simulink model "spiBitbang_MainClockDistr_v2_back"  (R2013b)
settings: Solver=FixedStepDiscrete  StartTime=0.0  StopTime=5e-4  FixedStep=Ts  RelTol=1e-3
model workspace (MAT data in the model file):
  Ts = 1e-06
undefined symbols (not defined in the file or in its folder): High, periSam, sampleTime, sigbuilder_block
libraries: simulink_extras x46, simulink x11, dspswit3 x8, dspsnks4 x1
settings Model: Creator=mainster  LastModifiedBy=mainster
settings ConfigurationSet: Description=SimMechanics 2G

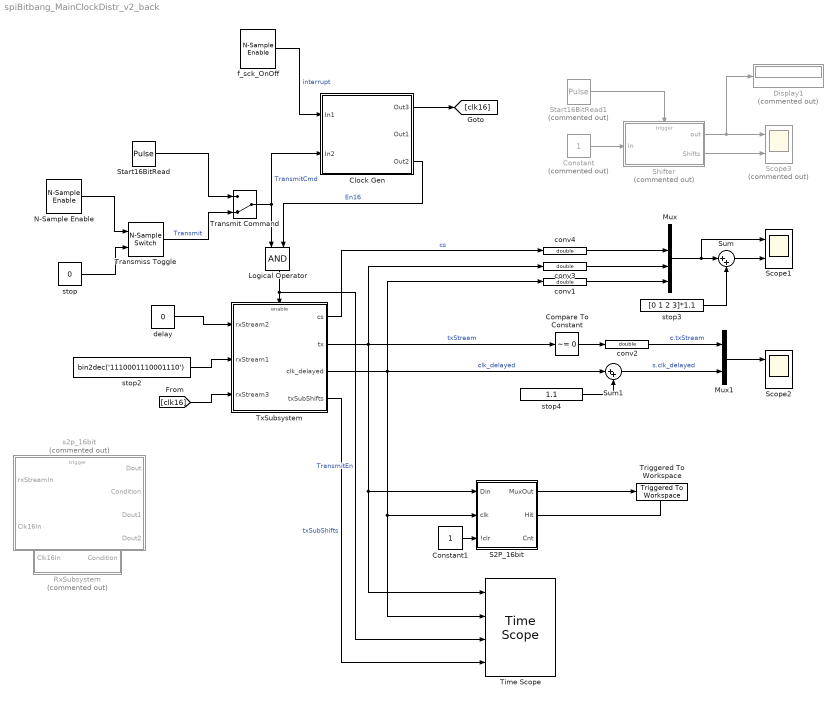
== system spiBitbang_MainClockDistr_v2_back ==
  Clock Gen : Subsystem
  Compare To Constant : simulink/Logic and Bit Operations/Compare To Constant  relop=~=  const=0  OutDataTypeStr=boolean
  Constant : Constant  Commented=on
  Constant1 : Constant  SampleTime=sampleTime
  Display1 : Display  Commented=on
  Logical Operator : Logic  AllPortsSameDT=off  OutDataTypeStr=boolean
  Mux : Mux
  Mux1 : Mux  Inputs=2
  N-Sample Enable : dspswit3/N-Sample Enable  N=20  ActiveLevel=High (1)  reset=off  TriggerType=Rising edge  Ts=-1  DataType=Logical
  RxSubsystem : Subsystem  Commented=on  TreatAsAtomicUnit=on
  S2P_16bit : Subsystem
  Scope1 : Scope  NumInputPorts=2
      settings: ShowLegends=on  TimeRange=0.0015  YMin=-0.2~-0.2  YMax=5~15
  Scope2 : Scope  NumInputPorts=2
      settings: ShowLegends=on  YMin=-0.2~-0.2  YMax=5~15  SaveName=ScopeData4
  Scope3 : Scope  Commented=on  NumInputPorts=2
      settings: ShowLegends=on  TimeRange=0.0015  YMin=-0.2~-0.2  YMax=5~15  SaveName=ScopeData3
  Shifter : Subsystem  Commented=on  TreatAsAtomicUnit=on
  Start16BitRead : DiscretePulseGenerator  Period=400  PulseWidth=35  PhaseDelay=20  SampleTime=Ts
  Start16BitRead1 : DiscretePulseGenerator  Commented=on  Period=100  PulseWidth=50  SampleTime=Ts
  Sum : Sum  Inputs=|++  LockScale=on
  Sum1 : Sum  Inputs=|++  LockScale=on
  Time Scope : TimeScope  NumInputPorts=4  DefaultConfigurationName=spbscopes.TimeScopeBlockCfg
      settings: CopyFcn=scopeextensions.ScopeBlock.onCoreBlockCopy(gcbh);  DeleteFcn=scopeextensions.ScopeBlock.callback(gcbh, 'onBlockDelete');  PreSaveFcn=scopeextensions.ScopeBlock.callback(gcbh, 'onModelSave');  NameChangeFcn=scopeextensions.ScopeBlock.callback(gcbh, 'onBlockRename');  DestroyFcn=scopeextensions.ScopeBlock.onBlockDestroy(gcbh)  CloseFcn=scopeextensions.ScopeBlock.callback(gcbh, 'onBlockClose');  PreDeleteFcn=scopeextensions.ScopeBlock.callback(gcbh, 'onBlockPreDelete');
  Transmiss Toggle : dspswit3/N-Sample Switch  N=250  reset=off  TriggerType=Rising edge  Ts=-1
  Transmit Command : ManualSwitch  CurrentSetting=0
  Triggered To Workspace : dspsnks4/Triggered To Workspace  TriggerType=Rising edge  VariableName=outDffShift  Buffer=1000  Save2DMode=2-D array (concatenate along first dimension)
      settings: FixptAsFi=off
  TxSubsystem : Subsystem
  conv{1..4} (4 alike) : DataTypeConversion  OutDataTypeStr=double  LockScale=on
  delay : Constant  Value=0  SampleTime=-1
  f_sck_OnOff : dspswit3/N-Sample Enable  N=1  ActiveLevel=High (1)  reset=off  TriggerType=Falling edge  Ts=-1  DataType=Boolean
  s2p_16bit : Subsystem  Commented=on
  stop : Constant  Value=0  OutDataTypeStr=Inherit: Inherit via back propagation  SampleTime=-1
  stop2 : Constant  Value=bin2dec('1110001110001110')  OutDataTypeStr=uint16  SampleTime=-1
  stop3 : Constant  Value=[0 1 2 3]*1.1  SampleTime=-1
  stop4 : Constant  Value=1.1  SampleTime=-1
  wires:
  f_sck_OnOff/1 -> Clock Gen/1(In1)  "interrupt"
  Sum/1 -> Scope1/2
  Mux/1 -> Scope1/1, Sum/1
  N-Sample Enable/1 -> Transmiss Toggle/1
  stop/1 -> Transmiss Toggle/2
  Transmit Command/1 -> Logical Operator/1, Clock Gen/2(In2)  "TransmitCmd"
  Transmiss Toggle/1 -> Transmit Command/2  "Transmit"
  Start16BitRead/1 -> Transmit Command/1
  Clock Gen/1(Out3) -> [clk16]
  delay/1 -> TxSubsystem/1(rxStream2)
  [clk16] -> TxSubsystem/3(rxStream3)
  stop2/1 -> TxSubsystem/2(rxStream1)
  stop3/1 -> Sum/2
  TxSubsystem/1(cs) -> conv4/1  "cs"
  conv1/1 -> Mux/4
  Start16BitRead1/1 -> Shifter/Trigger
  Constant/1 -> Shifter/1(In)
  Shifter/1(out) -> Display1/1, Scope3/1
  Shifter/2(Shifts) -> Scope3/2
  TxSubsystem/2(tx) -> Time Scope/1, S2P_16bit/1(Din), conv3/1, Compare To Constant/1  "txStream"
  TxSubsystem/3(clk_delayed) -> conv1/1, Time Scope/2, S2P_16bit/2(clk), Sum1/1  "clk_delayed"
  stop4/1 -> Sum1/2
  Sum1/1 -> Mux1/2  "s.clk_delayed"
  conv3/1 -> Mux/3
  conv4/1 -> Mux/2
  Compare To Constant/1 -> conv2/1
  Mux1/1 -> Scope2/1
  conv2/1 -> Mux1/1  "c.txStream"
  S2P_16bit/1(MuxOut) -> Triggered To Workspace/1
  Constant1/1 -> S2P_16bit/3(!clr)
  S2P_16bit/2(Hit) -> Triggered To Workspace/Trigger
  TxSubsystem/4(txSubShifts) -> Time Scope/4  "txSubShifts"
  Clock Gen/3(Out2) -> Logical Operator/2  "En16"
  Logical Operator/1 -> Time Scope/3, TxSubsystem/Enable  "TransmitEn"

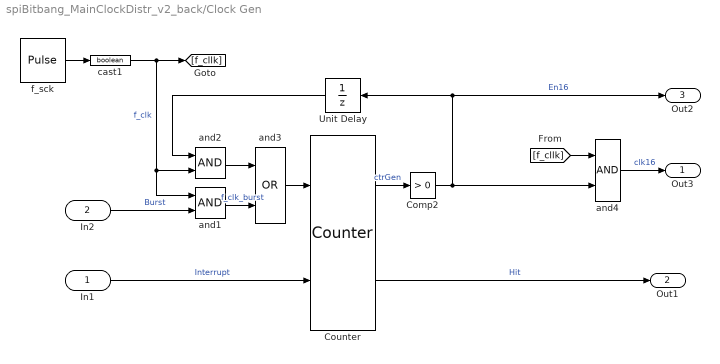
== system spiBitbang_MainClockDistr_v2_back/Clock Gen ==
  In1 : Inport
  In2 : Inport  Port=2
  Comp2 : simulink/Logic and Bit Operations/Compare To Constant  relop=>  const=0  OutDataTypeStr=boolean
  Counter : dspswit3/Counter  Direction=Up  CountEvent=Rising edge  CounterSize=User defined  MaxCount=16  InitialCount=0  Output=Count and Hit  HitValue=periSam/4  ResetInput=on  SamplesPerFrame=1  Ts=1  CntDtype=double  HitDtype=Logical
  Unit Delay : UnitDelay  SampleTime=-1
  and1 : Logic  AllPortsSameDT=off  OutDataTypeStr=boolean
      settings: AttributesFormatString=%<Tag>
  and2 : Logic  AllPortsSameDT=off  OutDataTypeStr=boolean
      settings: AttributesFormatString=%<Tag>
  and3 : Logic  Operator=OR  AllPortsSameDT=off  OutDataTypeStr=boolean
      settings: AttributesFormatString=%<Tag>
  and4 : Logic  AllPortsSameDT=off  OutDataTypeStr=boolean
      settings: AttributesFormatString=%<Tag>
  "cast1 " : DataTypeConversion  OutDataTypeStr=boolean
  f_sck : DiscretePulseGenerator  Period=periSam  PulseWidth=periSam/2  SampleTime=Ts
      settings: AttributesFormatString=|
      | Period =%<Period>
      | sTime=%<SampleTime>
      | Delay=%<PhaseDelay>
  Out3 : Outport
  Out1 : Outport  Port=2
  Out2 : Outport  Port=3
  wires:
  "cast1 "/1 -> and1/1, and2/2, [f_cllk]  "f_clk"
  f_sck/1 -> "cast1 "/1
  Comp2/1 -> Out2/1, Unit Delay/1, and4/2  "En16"
  Counter/1 -> Comp2/1  "ctrGen"
  In1/1 -> Counter/2  "Interrupt"
  In2/1 -> and1/2  "Burst"
  and3/1 -> Counter/1
  and4/1 -> Out3/1  "clk16"
  and1/1 -> and3/2  "f_clk_burst"
  and2/1 -> and3/1
  Unit Delay/1 -> and2/1
  Counter/2 -> Out1/1  "Hit"
  [f_cllk] -> and4/1

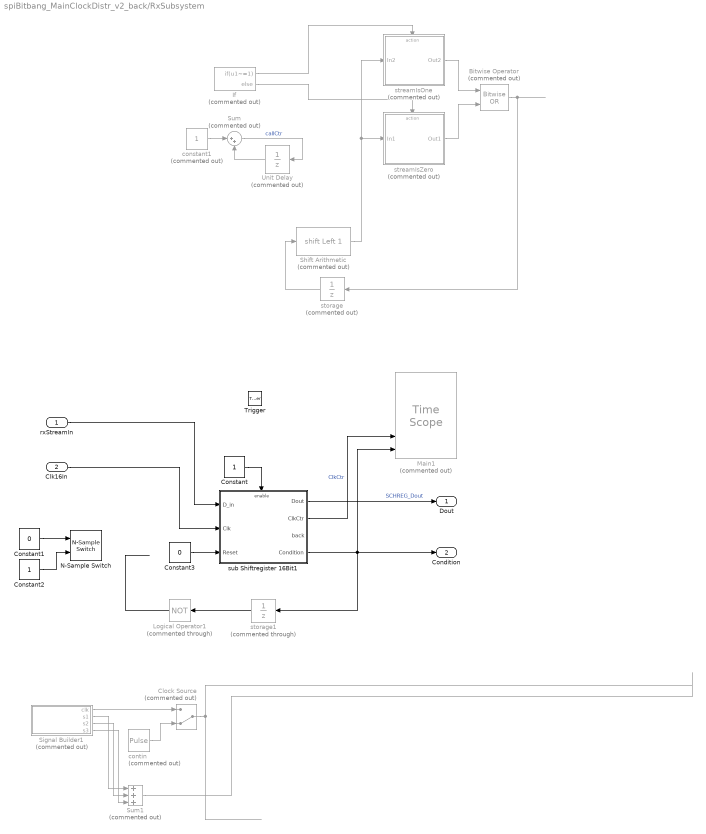
== system spiBitbang_MainClockDistr_v2_back/RxSubsystem ==
  rxStreamIn : Inport
  Clk16In : Inport  Port=2
  Trigger : TriggerPort
  Bitwise Operator : simulink/Logic and Bit Operations/Bitwise Operator  Commented=on  logicop=OR  UseBitMask=off  NumInputPorts=2  BitMask=bin2dec('11011001')  BitMaskRealWorld=Stored Integer
  Clock Source : ManualSwitch  Commented=on  CurrentSetting=0
  Constant : Constant
  Constant1 : Constant  Value=0  SampleTime=-1
  Constant2 : Constant  SampleTime=-1
  Constant3 : Constant  Value=0  SampleTime=-1
  If : If  Commented=on  IfExpression=u1~=1
  Logical Operator1 : Logic  Commented=through  Operator=NOT  IconShape=distinctive  AllPortsSameDT=off  OutDataTypeStr=boolean
  Main1 : TimeScope  Commented=on  NumInputPorts=6  DefaultConfigurationName=spbscopes.TimeScopeBlockCfg
      settings: CopyFcn=scopeextensions.ScopeBlock.onCoreBlockCopy(gcbh);  DeleteFcn=scopeextensions.ScopeBlock.callback(gcbh, 'onBlockDelete');  PreSaveFcn=scopeextensions.ScopeBlock.callback(gcbh, 'onModelSave');  NameChangeFcn=scopeextensions.ScopeBlock.callback(gcbh, 'onBlockRename');  DestroyFcn=scopeextensions.ScopeBlock.onBlockDestroy(gcbh)  CloseFcn=scopeextensions.ScopeBlock.callback(gcbh, 'onBlockClose');  PreDeleteFcn=scopeextensions.ScopeBlock.callback(gcbh, 'onBlockPreDelete');
  N-Sample Switch : dspswit3/N-Sample Switch  N=30  reset=off  TriggerType=Rising edge  Ts=-1
  Shift Arithmetic : ArithShift  Commented=on  BitShiftNumber=1  BitShiftDirection=Left  DiagnosticForOORShift=Warning  CheckOORBitShift=on
  Signal Builder1 : Subsystem  Tag=STV Subsys  Commented=on  LoadFcn=sigbuilder_block('load');  StartFcn=sigbuilder_block('start');  StopFcn=sigbuilder_block('stop');  ClipboardFcn=sigbuilder_block('clipboard');  TreatAsAtomicUnit=on  mask(Sigbuilder block){}
      mask help: Simulink:masks:SigbuilderBlock_MD
      mask init:
      | if ~strcmp(get_param(bdroot(gcbh),'SimulationStatus'),'stopped') tuvar = sigbuilder_block('maskInit'); end
      settings: CopyFcn=sigbuilder_block('copy');  DeleteFcn=sigbuilder_block('delete');  ModelCloseFcn=sigbuilder_block('modelClose');  PreSaveFcn=sigbuilder_block('preSave');  PauseFcn=sigbuilder_block('pause');  ContinueFcn=sigbuilder_block('continue');  NameChangeFcn=sigbuilder_block('namechange');  OpenFcn=sigbuilder_block('open',[367.5 149.25 803.25 388.5 ]);  CloseFcn=sigbuilder_block('close');
      mask Display: plot(0, 0, 100, 100,[2, 2, 32, 32, 2], [68, 8, 8, 68, 68],[32, 2], [38, 38], [32, 19, 2],[53, 60, 44], [32, 17, 17, 2],[16, 16, 31, 31]);txt = getActiveGroup(gcbh);text(2, 100, txt,'verticalAlignment', 'top');
  Sum : Sum  Commented=on  Inputs=|++  SaturateOnIntegerOverflow=on  InputSameDT=on  OutDataTypeStr=Inherit: Same as first input
  Sum1 : Sum  Commented=on  Inputs=+++  SampleTime=sampleTime
  Unit Delay : UnitDelay  Commented=on
  constant1 : Constant  Commented=on  OutDataTypeStr=int8  LockScale=on
  contin : DiscretePulseGenerator  Commented=on  Period=periSam  PulseWidth=periSam*0.5  SampleTime=sampleTime
  storage : UnitDelay  Commented=on  SampleTime=-1
  storage1 : UnitDelay  Commented=through  SampleTime=-1
  streamIsOne : Subsystem  Commented=on  TreatAsAtomicUnit=on
  streamIsZero : Subsystem  Commented=on  TreatAsAtomicUnit=on
  sub Shiftregister 16Bit1 : Subsystem  TreatAsAtomicUnit=on
  Dout : Outport
  Condition : Outport  Port=2
  wires:
  Sum/1 -> Unit Delay/1  "callCtr"
  constant1/1 -> Sum/1
  Unit Delay/1 -> Sum/2
  Shift Arithmetic/1 -> streamIsOne/1(In2), streamIsZero/1(In1)
  storage/1 -> Shift Arithmetic/1
  If/2 -> streamIsZero/Action
  If/1 -> streamIsOne/Action
  streamIsOne/1(Out2) -> Bitwise Operator/1
  streamIsZero/1(Out1) -> Bitwise Operator/2
  Bitwise Operator/1 -> storage/1
  sub Shiftregister 16Bit1/2(ClkCtr) -> Main1/5  "ClkCtr"
  sub Shiftregister 16Bit1/4(Condition) -> storage1/1, Condition/1, Main1/6
  rxStreamIn/1 -> sub Shiftregister 16Bit1/1(D_in)
  Signal Builder1/3(s2) -> Sum1/2
  Signal Builder1/2(s1) -> Sum1/1
  Signal Builder1/4(s3) -> Sum1/3
  Sum1/1 -> ?
  Clock Source/1 -> ?
  Signal Builder1/1(clk) -> Clock Source/1
  contin/1 -> Clock Source/2
  Clk16In/1 -> sub Shiftregister 16Bit1/2(Clk)
  Constant/1 -> sub Shiftregister 16Bit1/Enable
  Constant1/1 -> N-Sample Switch/1
  Constant2/1 -> N-Sample Switch/2
  Logical Operator1/1 -> ?
  sub Shiftregister 16Bit1/1(Dout) -> Dout/1  "SCHREG_Dout"
  storage1/1 -> Logical Operator1/1
  Constant3/1 -> sub Shiftregister 16Bit1/3(Reset)

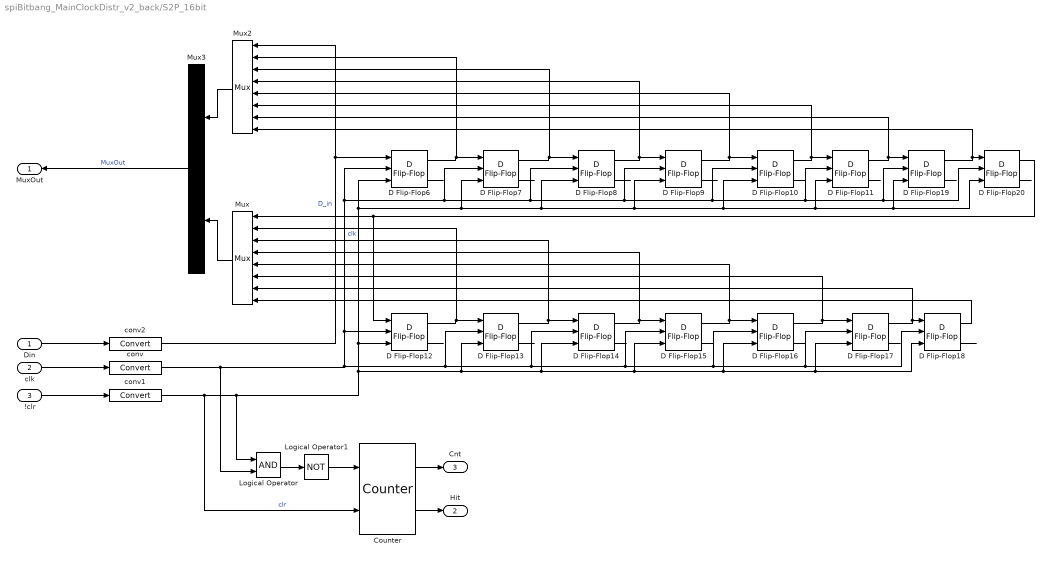
== system spiBitbang_MainClockDistr_v2_back/S2P_16bit ==
  Din : Inport
  clk : Inport  Port=2
  !clr : Inport  Port=3
  Counter : dspswit3/Counter  Direction=Up  CountEvent=Falling edge  CounterSize=User defined  MaxCount=16  InitialCount=0  Output=Count and Hit  HitValue=8  ResetInput=on  SamplesPerFrame=1  Ts=1  CntDtype=double  HitDtype=Logical
  D Flip-Flop{6..20} (15 alike) : simulink_extras/Flip Flops/D Flip-Flop
  Logical Operator : Logic  AllPortsSameDT=off  OutDataTypeStr=boolean
  Logical Operator1 : Logic  Operator=NOT  IconShape=distinctive  AllPortsSameDT=off  OutDataTypeStr=boolean
  Mux : Mux  Inputs=8
  Mux2 : Mux  Inputs=8
  Mux3 : Mux  Inputs=2
  conv : DataTypeConversion
  conv1 : DataTypeConversion
  conv2 : DataTypeConversion
  MuxOut : Outport
  Hit : Outport  Port=2
  Cnt : Outport  Port=3
  wires:
  D Flip-Flop7/1 -> Mux2/3, D Flip-Flop8/1
  D Flip-Flop13/1 -> Mux/3, D Flip-Flop14/1
  D Flip-Flop16/1 -> Mux/6, D Flip-Flop17/1
  D Flip-Flop17/1 -> Mux/7, D Flip-Flop18/1
  D Flip-Flop11/1 -> Mux2/7, D Flip-Flop19/1
  conv2/1 -> D Flip-Flop6/1, Mux2/1  "D_in"
  D Flip-Flop8/1 -> Mux2/4, D Flip-Flop9/1
  D Flip-Flop10/1 -> Mux2/6, D Flip-Flop11/1
  D Flip-Flop14/1 -> Mux/4, D Flip-Flop15/1
  D Flip-Flop18/1 -> Mux/8
  D Flip-Flop6/1 -> Mux2/2, D Flip-Flop7/1
  D Flip-Flop9/1 -> Mux2/5, D Flip-Flop10/1
  D Flip-Flop15/1 -> Mux/5, D Flip-Flop16/1
  Mux/1 -> Mux3/2
  D Flip-Flop12/1 -> Mux/2, D Flip-Flop13/1
  Mux3/1 -> MuxOut/1  "MuxOut"
  conv1/1 -> Counter/2, Logical Operator/1, D Flip-Flop6/3, D Flip-Flop19/3, D Flip-Flop20/3, D Flip-Flop11/3, D Flip-Flop10/3, D Flip-Flop9/3, D Flip-Flop8/3, D Flip-Flop7/3, D Flip-Flop12/3, D Flip-Flop18/3, D Flip-Flop17/3, D Flip-Flop16/3, D Flip-Flop15/3, D Flip-Flop14/3, D Flip-Flop13/3  "clr"
  D Flip-Flop20/1 -> D Flip-Flop12/1, Mux/1
  Mux2/1 -> Mux3/1
  D Flip-Flop19/1 -> Mux2/8, D Flip-Flop20/1
  conv/1 -> Logical Operator/2, D Flip-Flop6/2, D Flip-Flop20/2, D Flip-Flop19/2, D Flip-Flop11/2, D Flip-Flop10/2, D Flip-Flop9/2, D Flip-Flop8/2, D Flip-Flop7/2, D Flip-Flop12/2, D Flip-Flop13/2, D Flip-Flop16/2, D Flip-Flop17/2, D Flip-Flop18/2, D Flip-Flop15/2, D Flip-Flop14/2  "clk"
  D Flip-Flop15/2 -> ?
  D Flip-Flop14/2 -> ?
  D Flip-Flop18/2 -> ?
  D Flip-Flop19/2 -> ?
  D Flip-Flop20/2 -> ?
  D Flip-Flop17/2 -> ?
  D Flip-Flop13/2 -> ?
  D Flip-Flop6/2 -> ?
  D Flip-Flop11/2 -> ?
  !clr/1 -> conv1/1
  D Flip-Flop8/2 -> ?
  D Flip-Flop9/2 -> ?
  D Flip-Flop7/2 -> ?
  D Flip-Flop16/2 -> ?
  D Flip-Flop12/2 -> ?
  D Flip-Flop10/2 -> ?
  clk/1 -> conv/1
  Din/1 -> conv2/1
  Logical Operator/1 -> Logical Operator1/1
  Logical Operator1/1 -> Counter/1
  Counter/1 -> Cnt/1
  Counter/2 -> Hit/1

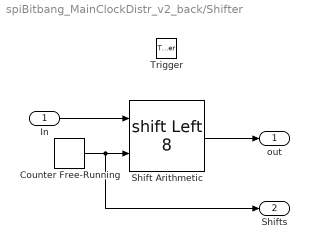
== system spiBitbang_MainClockDistr_v2_back/Shifter ==
  In : Inport
  Trigger : TriggerPort  PortDimensions=1
  Counter Free-Running : simulink/Sources/Counter Free-Running  NumBits=3  tsamp=-1
  Shift Arithmetic : ArithShift  BitShiftNumberSource=Input port  BitShiftNumber=8  BitShiftDirection=Left
      settings: InputPortMap=u0,p1
  out : Outport
  Shifts : Outport  Port=2
  wires:
  Shift Arithmetic/1 -> out/1
  In/1 -> Shift Arithmetic/1
  Counter Free-Running/1 -> Shifts/1, Shift Arithmetic/2

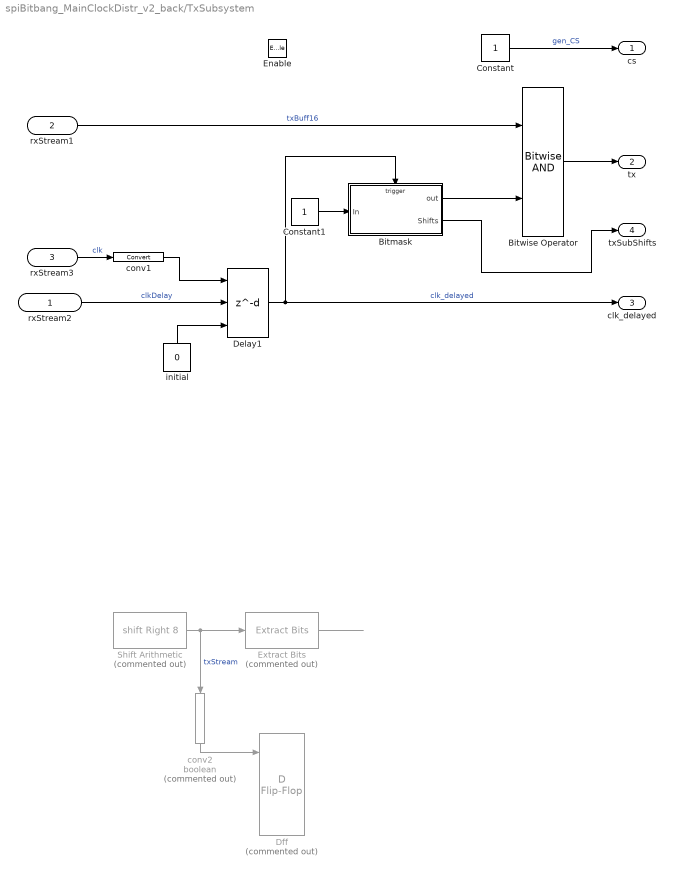
== system spiBitbang_MainClockDistr_v2_back/TxSubsystem ==
  rxStream2 : Inport
  rxStream1 : Inport  Port=2  OutDataTypeStr=uint16
  rxStream3 : Inport  Port=3
  Enable : EnablePort  StatesWhenEnabling=reset
  Bitmask : Subsystem  TreatAsAtomicUnit=on
  Bitwise Operator : simulink/Logic and Bit Operations/Bitwise Operator  logicop=AND  UseBitMask=off  NumInputPorts=2  BitMask=bin2dec('11011001')  BitMaskRealWorld=Stored Integer
  Constant : Constant  SampleTime=-1
  Constant1 : Constant
  Delay1 : Delay  DelayLengthSource=Input port  DelayLength=1  InitialConditionSource=Input port  InitialCondition=0  InputProcessing=Inherited
      settings: InputPortMap=u0,p1,p4
  Dff : simulink_extras/Flip Flops/D Flip-Flop  Commented=on
  Extract Bits : simulink/Logic and Bit Operations/Extract Bits  Commented=on  bitsToExtract=Range of bits  numBits=8  bitIdxRange=0  outScalingMode=Preserve fixed-point scaling
  Shift Arithmetic : ArithShift  Commented=on  BitShiftNumberSource=Input port  BitShiftNumber=8  BitShiftDirection=Right  CheckOORBitShift=on
      settings: InputPortMap=u0,p1
  conv1 : DataTypeConversion
  conv2 : DataTypeConversion  Commented=on  OutDataTypeStr=boolean  LockScale=on
  initial : Constant  Value=0  SampleTime=-1
  cs : Outport  InitialOutput=1
  tx : Outport  Port=2  InitialOutput=1
  clk_delayed : Outport  Port=3  InitialOutput=1
  txSubShifts : Outport  Port=4  InitialOutput=1
  wires:
  rxStream2/1 -> Delay1/2  "clkDelay"
  initial/1 -> Delay1/3
  Constant/1 -> cs/1  "gen_CS"
  rxStream1/1 -> Bitwise Operator/1  "txBuff16"
  rxStream3/1 -> conv1/1  "clk"
  Delay1/1 -> clk_delayed/1, Bitmask/Trigger  "clk_delayed"
  conv1/1 -> Delay1/1
  Constant1/1 -> Bitmask/1(In)
  Shift Arithmetic/1 -> conv2/1, Extract Bits/1  "txStream"
  conv2/1 -> Dff/1
  Extract Bits/1 -> ?
  Bitmask/1(out) -> Bitwise Operator/2
  Bitwise Operator/1 -> tx/1
  Bitmask/2(Shifts) -> txSubShifts/1

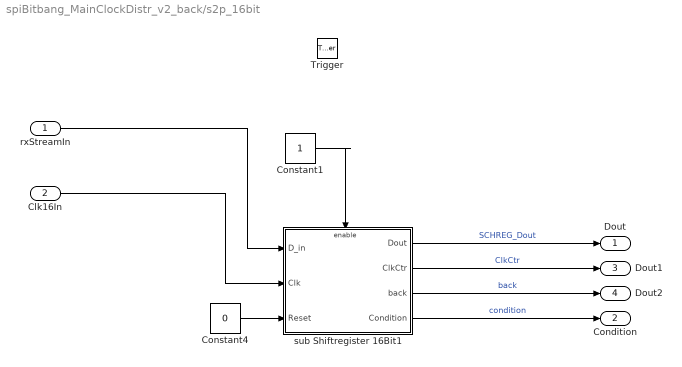
== system spiBitbang_MainClockDistr_v2_back/s2p_16bit ==
  rxStreamIn : Inport
  Clk16In : Inport  Port=2
  Trigger : TriggerPort  PortDimensions=1
  Constant1 : Constant
  Constant4 : Constant  Value=0  SampleTime=-1
  sub Shiftregister 16Bit1 : Subsystem  TreatAsAtomicUnit=on
  Dout : Outport
  Condition : Outport  Port=2
  Dout1 : Outport  Port=3
  Dout2 : Outport  Port=4
  wires:
  sub Shiftregister 16Bit1/4(Condition) -> Condition/1  "condition"
  rxStreamIn/1 -> sub Shiftregister 16Bit1/1(D_in)
  Clk16In/1 -> sub Shiftregister 16Bit1/2(Clk)
  sub Shiftregister 16Bit1/1(Dout) -> Dout/1  "SCHREG_Dout"
  Constant4/1 -> sub Shiftregister 16Bit1/3(Reset)
  sub Shiftregister 16Bit1/2(ClkCtr) -> Dout1/1  "ClkCtr"
  sub Shiftregister 16Bit1/3(back) -> Dout2/1  "back"
  Constant1/1 -> sub Shiftregister 16Bit1/Enable

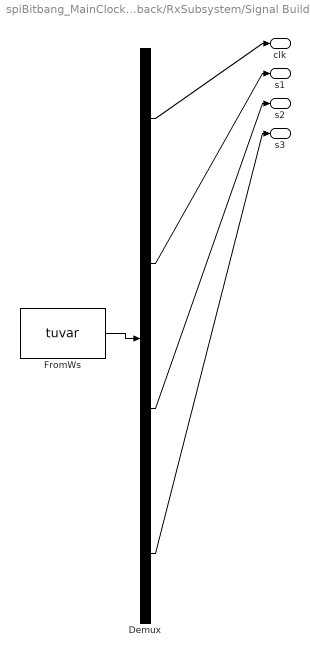
== system spiBitbang_MainClockDistr_v2_back/RxSubsystem/Signal Builder1 ==
  Demux : Demux  Tag=STV Demux
  FromWs : FromWorkspace  Tag=STV FromWs  VariableName=tuvar  SampleTime=0
      SigBuilderData=|
      | common.afterFinalStr = 'Extrapolate'
      | common.sampleTime = '0'
      | dataSet.timeRange = [0 0.00032]
      | dataSet.name = 'Group 1'
      | sbobj.Groups.Name = 'Group 1'
      | sbobj.Groups.Signals(1).Name = 'clk'
      | sbobj.Groups.Signals(1).XData = [0 1e-05 1e-05 2e-05 2e-05 3e-05 3e-05 4e-05 4e-05 5e-05 5e-05 6e-05 6e-05 7e-05 7e-05 8e-05 8e-05 9e-05 9e-05 0.0001 0.0001 0.00011 0.00011 0.00012 0.00012 0.00013 0.00013 0.00014 0.00014 0.00015 0.00015 0.00016 0.00016 0.00017 0.00017 0.00018 0.00018 0.00019 0.00019 0.0002 0.0002 0.00021 0.00021 0.00022 0.00022 0.00023 0.00023 0.00024 0.00024 0.00025 0.00025 0.00026 0.00026 0.00027 0.00027 0.00028 0.00028 0.00029 0.00029 0.0003 0.0003 0.00031 0.00031 0.00032]
      | sbobj.Groups.Signals(1).YData = [1 1 0 0 1 1 0 0 1 1 0 0 1 1 0 0 1 1 0 0 1 1 0 0 1 1 0 0 1 1 0 0 1 1 0 0 1 1 0 0 1 1 0 0 1 1 0 0 1 1 0 0 1 1 0 0 1 1 0 0 1 1 0 0]
      | sbobj.Groups.Signals(2).Name = 's1'
      | sbobj.Groups.Signals(2).XData = [0 5e-06 5e-06 5.45e-05 5.45e-05 0.00032]
      | sbobj.Groups.Signals(2).YData = [0 0 1 1 0 0]
      | sbobj.Groups.Signals(3).Name = 's2'
      | sbobj.Groups.Signals(3).XData = [0 0.0001475 0.0001475 0.000196 0.000196 0.00032]
      | sbobj.Groups.Signals(3).YData = [0 0 1 1 0 0]
      | sbobj.Groups.Signals(4).Name = 's3'
      | sbobj.Groups.Signals(4).XData = [0 0.000237 0.000237 0.000297 0.000297 0.00032]
      | sbobj.Groups.Signals(4).YData = [0 0 1 1 0 0]
      | sbobj.Groups.TimeRange = [0 0.00032]
  clk : Outport  Tag=STV Outport
  s1 : Outport  Tag=STV Outport  Port=2
  s2 : Outport  Tag=STV Outport  Port=3
  s3 : Outport  Tag=STV Outport  Port=4
  wires:
  FromWs/1 -> Demux/1
  Demux/1 -> clk/1
  Demux/2 -> s1/1
  Demux/3 -> s2/1
  Demux/4 -> s3/1

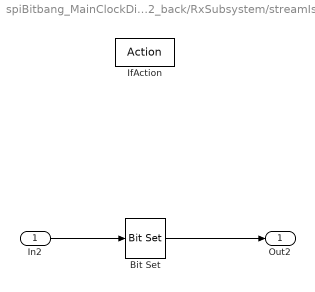
== system spiBitbang_MainClockDistr_v2_back/RxSubsystem/streamIsOne ==
  In2 : Inport  OutDataTypeStr=int8
  IfAction : ActionPort
  Bit Set : simulink/Logic and Bit Operations/Bit Set  iBit=0
  Out2 : Outport  OutDataTypeStr=uint8
  wires:
  In2/1 -> Bit Set/1
  Bit Set/1 -> Out2/1

== system spiBitbang_MainClockDistr_v2_back/RxSubsystem/streamIsZero ==
  In1 : Inport  OutDataTypeStr=int8
  IfAction : ActionPort
  Bit Clear : simulink/Logic and Bit Operations/Bit Clear  iBit=0
  Out1 : Outport  OutDataTypeStr=uint8
  wires:
  In1/1 -> Bit Clear/1
  Bit Clear/1 -> Out1/1

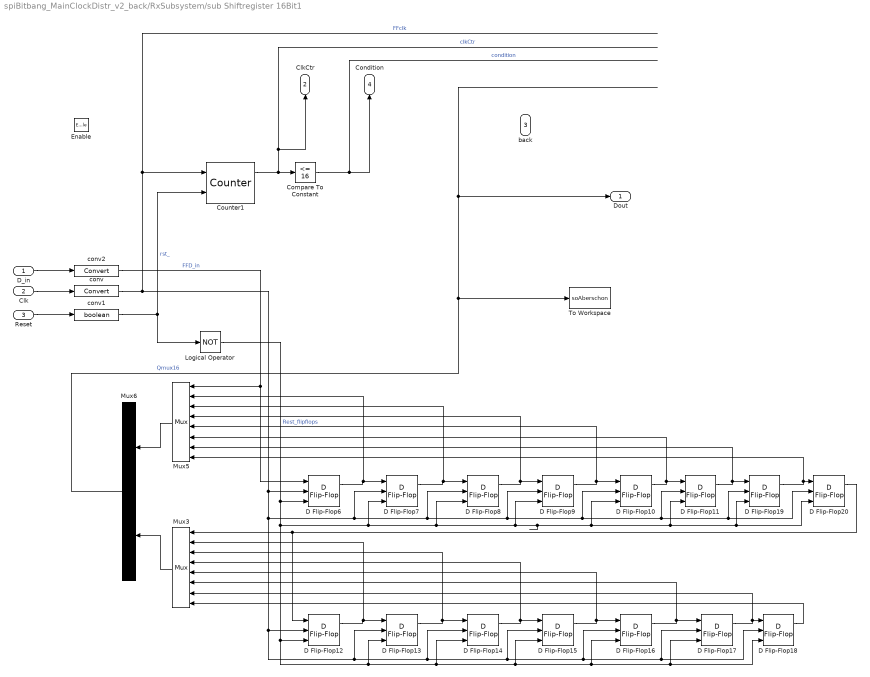
== system spiBitbang_MainClockDistr_v2_back/RxSubsystem/sub Shiftregister 16Bit1 ==
  D_in : Inport
  Clk : Inport  Port=2
  Reset : Inport  Port=3
  Enable : EnablePort  StatesWhenEnabling=reset
  Compare To Constant : simulink/Logic and Bit Operations/Compare To Constant  relop=<=  const=16  OutDataTypeStr=boolean  ZeroCross=off
  Counter1 : dspswit3/Counter  Direction=Up  CountEvent=Rising edge  CounterSize=User defined  MaxCount=255  InitialCount=0  Output=Count and Hit  HitValue=32  ResetInput=on  SamplesPerFrame=1  Ts=1  CntDtype=double  HitDtype=Boolean
  D Flip-Flop{6..20} (15 alike) : simulink_extras/Flip Flops/D Flip-Flop
  Logical Operator : Logic  Operator=NOT  IconShape=distinctive  AllPortsSameDT=off  OutDataTypeStr=boolean
  Mux3 : Mux  Inputs=8
  Mux5 : Mux  Inputs=8
  Mux6 : Mux  Inputs=2
  To Workspace : ToWorkspace  VariableName=soAberschon  SampleTime=-1  SaveFormat=Timeseries
  conv : DataTypeConversion  LockScale=on
  conv1 : DataTypeConversion  OutDataTypeStr=boolean
  conv2 : DataTypeConversion
  Dout : Outport
  ClkCtr : Outport  Port=2
  back : Outport  Port=3
  Condition : Outport  Port=4
  wires:
  D Flip-Flop6/1 -> Mux5/2, D Flip-Flop7/1
  D Flip-Flop7/1 -> Mux5/3, D Flip-Flop8/1
  D Flip-Flop9/1 -> Mux5/5, D Flip-Flop10/1
  D Flip-Flop10/1 -> Mux5/6, D Flip-Flop11/1
  D Flip-Flop12/1 -> Mux3/2, D Flip-Flop13/1
  D Flip-Flop13/1 -> Mux3/3, D Flip-Flop14/1
  D Flip-Flop14/1 -> Mux3/4, D Flip-Flop15/1
  D Flip-Flop17/1 -> Mux3/7, D Flip-Flop18/1
  conv/1 -> D Flip-Flop13/2, D Flip-Flop16/2, D Flip-Flop17/2, D Flip-Flop18/2, D Flip-Flop15/2, D Flip-Flop14/2, D Flip-Flop12/2, D Flip-Flop20/2, D Flip-Flop19/2, D Flip-Flop11/2, D Flip-Flop10/2, D Flip-Flop9/2, D Flip-Flop8/2, D Flip-Flop7/2, D Flip-Flop6/2, Counter1/1  "FFclk"
  D Flip-Flop8/1 -> Mux5/4, D Flip-Flop9/1
  D Flip-Flop15/1 -> Mux3/5, D Flip-Flop16/1
  D Flip-Flop16/1 -> Mux3/6, D Flip-Flop17/1
  D Flip-Flop18/1 -> Mux3/8
  D Flip-Flop19/1 -> Mux5/8, D Flip-Flop20/1
  D Flip-Flop11/1 -> Mux5/7, D Flip-Flop19/1
  D Flip-Flop20/1 -> D Flip-Flop12/1, Mux3/1
  conv2/1 -> D Flip-Flop6/1, Mux5/1  "FFD_in"
  Mux5/1 -> Mux6/1
  Mux3/1 -> Mux6/2
  D_in/1 -> conv2/1
  Clk/1 -> conv/1
  Counter1/1 -> ClkCtr/1, Compare To Constant/1  "clkCtr"
  Compare To Constant/1 -> Condition/1  "condition"
  conv1/1 -> Logical Operator/1, Counter1/2  "rst_"
  Reset/1 -> conv1/1
  Logical Operator/1 -> D Flip-Flop6/3, D Flip-Flop18/3, D Flip-Flop17/3, D Flip-Flop16/3, D Flip-Flop15/3, D Flip-Flop14/3, D Flip-Flop13/3, D Flip-Flop12/3, D Flip-Flop19/3, D Flip-Flop20/3, D Flip-Flop11/3, D Flip-Flop10/3, D Flip-Flop9/3, D Flip-Flop8/3, D Flip-Flop7/3  "Rest_flipflops"
  Mux6/1 -> To Workspace/1, Dout/1  "Qmux16"

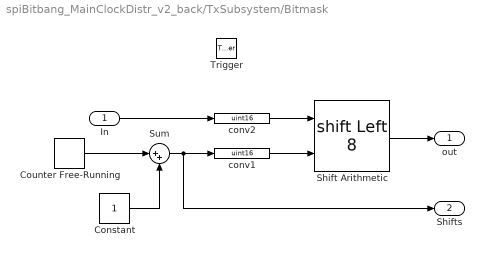
== system spiBitbang_MainClockDistr_v2_back/TxSubsystem/Bitmask ==
  In : Inport
  Trigger : TriggerPort  PortDimensions=1
  Constant : Constant  SampleTime=-1
  Counter Free-Running : simulink/Sources/Counter Free-Running  NumBits=15  tsamp=-1
  Shift Arithmetic : ArithShift  BitShiftNumberSource=Input port  BitShiftNumber=8  BitShiftDirection=Left
      settings: InputPortMap=u0,p1
  Sum : Sum  Inputs=|++
  conv1 : DataTypeConversion  OutDataTypeStr=uint16
  conv2 : DataTypeConversion  OutDataTypeStr=uint16
  out : Outport
  Shifts : Outport  Port=2
  wires:
  Shift Arithmetic/1 -> out/1
  In/1 -> conv2/1
  Counter Free-Running/1 -> Sum/1
  Sum/1 -> Shifts/1, conv1/1
  Constant/1 -> Sum/2
  conv1/1 -> Shift Arithmetic/2
  conv2/1 -> Shift Arithmetic/1

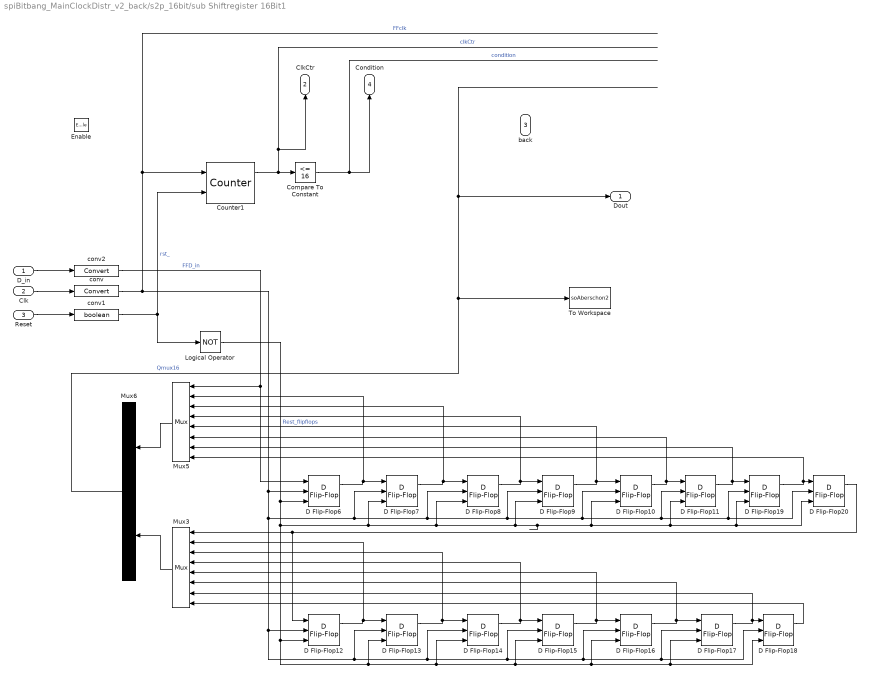
== system spiBitbang_MainClockDistr_v2_back/s2p_16bit/sub Shiftregister 16Bit1 ==
  D_in : Inport
  Clk : Inport  Port=2
  Reset : Inport  Port=3
  Enable : EnablePort  StatesWhenEnabling=reset
  Compare To Constant : simulink/Logic and Bit Operations/Compare To Constant  relop=<=  const=16  OutDataTypeStr=boolean  ZeroCross=off
  Counter1 : dspswit3/Counter  Direction=Up  CountEvent=Rising edge  CounterSize=User defined  MaxCount=255  InitialCount=0  Output=Count and Hit  HitValue=32  ResetInput=on  SamplesPerFrame=1  Ts=1  CntDtype=double  HitDtype=Boolean
  D Flip-Flop{6..20} (15 alike) : simulink_extras/Flip Flops/D Flip-Flop
  Logical Operator : Logic  Operator=NOT  IconShape=distinctive  AllPortsSameDT=off  OutDataTypeStr=boolean
  Mux3 : Mux  Inputs=8
  Mux5 : Mux  Inputs=8
  Mux6 : Mux  Inputs=2
  To Workspace : ToWorkspace  VariableName=soAberschon2  SampleTime=-1  SaveFormat=Timeseries
  conv : DataTypeConversion  LockScale=on
  conv1 : DataTypeConversion  OutDataTypeStr=boolean
  conv2 : DataTypeConversion
  Dout : Outport
  ClkCtr : Outport  Port=2
  back : Outport  Port=3
  Condition : Outport  Port=4
  wires:
  D Flip-Flop6/1 -> Mux5/2, D Flip-Flop7/1
  D Flip-Flop7/1 -> Mux5/3, D Flip-Flop8/1
  D Flip-Flop9/1 -> Mux5/5, D Flip-Flop10/1
  D Flip-Flop10/1 -> Mux5/6, D Flip-Flop11/1
  D Flip-Flop12/1 -> Mux3/2, D Flip-Flop13/1
  D Flip-Flop13/1 -> Mux3/3, D Flip-Flop14/1
  D Flip-Flop14/1 -> Mux3/4, D Flip-Flop15/1
  D Flip-Flop17/1 -> Mux3/7, D Flip-Flop18/1
  conv/1 -> D Flip-Flop13/2, D Flip-Flop16/2, D Flip-Flop17/2, D Flip-Flop18/2, D Flip-Flop15/2, D Flip-Flop14/2, D Flip-Flop12/2, D Flip-Flop20/2, D Flip-Flop19/2, D Flip-Flop11/2, D Flip-Flop10/2, D Flip-Flop9/2, D Flip-Flop8/2, D Flip-Flop7/2, D Flip-Flop6/2, Counter1/1  "FFclk"
  D Flip-Flop8/1 -> Mux5/4, D Flip-Flop9/1
  D Flip-Flop15/1 -> Mux3/5, D Flip-Flop16/1
  D Flip-Flop16/1 -> Mux3/6, D Flip-Flop17/1
  D Flip-Flop18/1 -> Mux3/8
  D Flip-Flop19/1 -> Mux5/8, D Flip-Flop20/1
  D Flip-Flop11/1 -> Mux5/7, D Flip-Flop19/1
  D Flip-Flop20/1 -> D Flip-Flop12/1, Mux3/1
  conv2/1 -> D Flip-Flop6/1, Mux5/1  "FFD_in"
  Mux5/1 -> Mux6/1
  Mux3/1 -> Mux6/2
  D_in/1 -> conv2/1
  Clk/1 -> conv/1
  Counter1/1 -> ClkCtr/1, Compare To Constant/1  "clkCtr"
  Compare To Constant/1 -> Condition/1  "condition"
  conv1/1 -> Logical Operator/1, Counter1/2  "rst_"
  Reset/1 -> conv1/1
  Logical Operator/1 -> D Flip-Flop6/3, D Flip-Flop18/3, D Flip-Flop17/3, D Flip-Flop16/3, D Flip-Flop15/3, D Flip-Flop14/3, D Flip-Flop13/3, D Flip-Flop12/3, D Flip-Flop19/3, D Flip-Flop20/3, D Flip-Flop11/3, D Flip-Flop10/3, D Flip-Flop9/3, D Flip-Flop8/3, D Flip-Flop7/3  "Rest_flipflops"
  Mux6/1 -> To Workspace/1, Dout/1  "Qmux16"
